simulink model "mrsRobotDetectorModel"  (R2018a)
settings: Solver=VariableStepAuto  StartTime=0.0  StopTime=10.0  RelTol=1e-3
libraries: mobileRoboticsLib x5
settings Model: Creator=scastro  LastModifiedBy=scastro

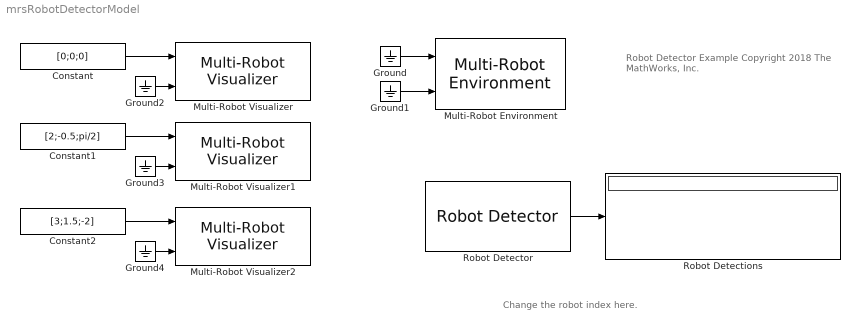
== system mrsRobotDetectorModel ==
  note: Change the robot index here.
  note: Robot Detector Example
      |
      | Copyright 2018 The MathWorks, Inc.
  Constant : Constant  Value=[0;0;0]
  Constant1 : Constant  Value=[2;-0.5;pi/2]
  Constant2 : Constant  Value=[3;1.5;-2]
  Ground{,1..4} (5 alike) : Ground
  Multi-Robot Environment : mobileRoboticsLib/Environments/Multi-Robot Environment  numRobots=3
      settings: SourceProductName=Mobile Robotics Simulation Toolbox
  Multi-Robot Visualizer : mobileRoboticsLib/Environments/Multi-Robot Visualizer  idx=1  radius=0  showTraj=off  hasLidar=off  sensorOffset=[ 0, 0 ]  scanAngles=[ -pi/4, 0, pi/4 ]  hasObjDetector=off  objDetectorOffset=[ 0, 0 ]  objDetectorAngle=0  objDetectorFOV=pi/3  objDetectorMaxRange=5
      settings: SourceProductName=Mobile Robotics Simulation Toolbox
  Multi-Robot Visualizer1 : mobileRoboticsLib/Environments/Multi-Robot Visualizer  idx=2  radius=0  showTraj=off  hasLidar=off  sensorOffset=[ 0, 0 ]  scanAngles=[ -pi/4, 0, pi/4 ]  hasObjDetector=off  objDetectorOffset=[ 0, 0 ]  objDetectorAngle=0  objDetectorFOV=pi/3  objDetectorMaxRange=5
      settings: SourceProductName=Mobile Robotics Simulation Toolbox
  Multi-Robot Visualizer2 : mobileRoboticsLib/Environments/Multi-Robot Visualizer  idx=3  radius=0  showTraj=off  hasLidar=off  sensorOffset=[ 0, 0 ]  scanAngles=[ -pi/4, 0, pi/4 ]  hasObjDetector=off  objDetectorOffset=[ 0, 0 ]  objDetectorAngle=0  objDetectorFOV=pi/3  objDetectorMaxRange=5
      settings: SourceProductName=Mobile Robotics Simulation Toolbox
  Robot Detections : Display
  Robot Detector : mobileRoboticsLib/Environments/Robot Detector  robotIdx=1  sensorOffset=[ 0, 0 ]  sensorAngle=0  fieldOfView=pi/2  maxRange=5  maxDetections=3  sampleTime=0.1
      settings: SourceProductName=Mobile Robotics Simulation Toolbox
  wires:
  Ground/1 -> Multi-Robot Environment/1
  Ground1/1 -> Multi-Robot Environment/2
  Robot Detector/1 -> Robot Detections/1
  Ground2/1 -> Multi-Robot Visualizer/2
  Ground3/1 -> Multi-Robot Visualizer1/2
  Ground4/1 -> Multi-Robot Visualizer2/2
  Constant/1 -> Multi-Robot Visualizer/1
  Constant1/1 -> Multi-Robot Visualizer1/1
  Constant2/1 -> Multi-Robot Visualizer2/1
